simulink model "InvertedPendulumNoise"  (Simulink 7.5)
settings: Solver=ode45  SolverMode=SingleTasking  StartTime=0.0  StopTime=10  RelTol=1e-3  AbsTol=1e-6
values from neighbouring files (symbols this model uses):
  b = 0.1    [IP_BODE.m]    (also in IP_DIS.m; IP_FDT.m; IP_PID_1.m; IP_PID_2.m)
  g = 9.8    [IP_BODE.m]    (also in IP_DIS.m; IP_FDT.m; IP_PID_1.m; IP_PID_2.m)
  i = 0.006    [IP_BODE.m]    (also in IP_DIS.m; IP_FDT.m; IP_PID_1.m; IP_PID_2.m)
  l = 0.3    [IP_BODE.m]    (also in IP_DIS.m; IP_FDT.m; IP_PID_1.m; IP_PID_2.m)
  M = .5    (= 0.5)    [IP_BODE.m]    (also in IP_DIS.m; IP_FDT.m; IP_PID_1.m; IP_PID_2.m)
  m = 0.2    [IP_BODE.m]    (also in IP_DIS.m; IP_FDT.m; IP_PID_1.m; IP_PID_2.m)
libraries: simulink_need_slupdate x1
settings Model: Creator=neoben  LastModifiedBy=neoben
settings DataIOCC: LimitDataPoints=off
settings OptimizationCC: BlockReduction=off  BooleanDataType=off
settings DebuggingCC: SaveWithParameterizedLinksMsg=none  SignalResolutionControl=TryResolveAllWithWarning  SolverPrmCheckMsg=none  MultiTaskDSMMsg=warning  MultiTaskCondExecSysMsg=none  StrictBusMsg=None
settings HardwareCC: TargetUnknown=on
settings RTWCC: IncludeERTFirstTime=on

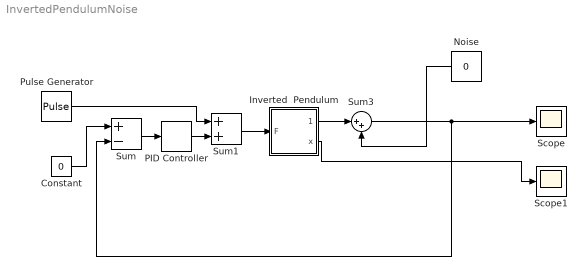
== system InvertedPendulumNoise ==
  Constant : Constant  Value=0
  Inverted  Pendulum : Subsystem
  Noise : Constant  Value=0  OutDataType=fixdt(1, 16)  OutScaling=2^0
  PID Controller : simulink_need_slupdate/PID Controller  SystemSampleTime=-1  P=100  I=1  D=20
  Pulse Generator : DiscretePulseGenerator  PulseType=Time based  Amplitude=1000  Period=10  PulseWidth=.01  PhaseDelay=0  SampleTime=1
  Scope : Scope
      settings: TickLabels=on  YMin=0  YMax=0.045  DataFormat=Array  MaxDataPoints=7000
  Scope1 : Scope
      settings: TickLabels=on  DataFormat=Array
  Sum : Sum  Inputs=+-  SaturateOnIntegerOverflow=on  InputSameDT=on  OutDataTypeStr=Inherit: Same as first input
  Sum1 : Sum  SaturateOnIntegerOverflow=on  InputSameDT=on  OutDataTypeStr=Inherit: Same as first input
  Sum3 : Sum  Inputs=|++  OutDataType=fixdt(1, 16)  OutScaling=2^0
  wires:
  Sum/1 -> PID Controller/1
  PID Controller/1 -> Sum1/2
  Inverted  Pendulum/1(Theta) -> Sum3/1
  Constant/1 -> Sum/1
  Pulse Generator/1 -> Sum1/1
  Sum1/1 -> Inverted  Pendulum/1(F)
  Inverted  Pendulum/2(x) -> Scope1/1
  Noise/1 -> Sum3/2
  Sum3/1 -> Sum/2, Scope/1

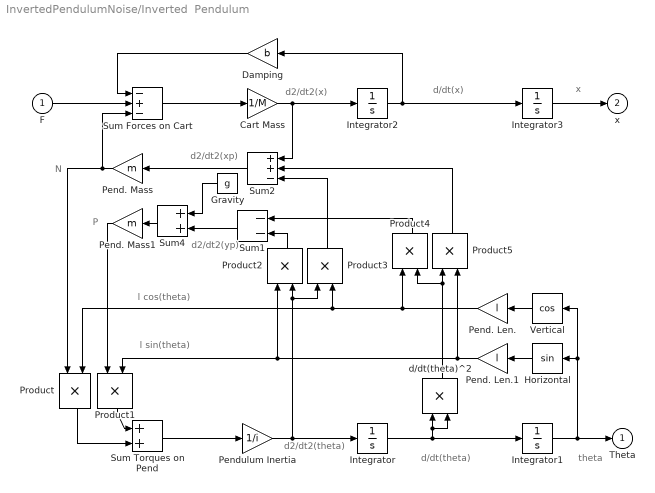
== system InvertedPendulumNoise/Inverted  Pendulum ==
  note: d2/dt2(xp)
  note: d2/dt2(yp)
  note: P
  note: N
  note: l sin(theta)
  note: l cos(theta)
  note: x
  note: d/dt(x)
  note: d2/dt2(x)
  note: d2/dt2(theta)
  note: d/dt(theta)
  note: theta
  F : Inport
  Cart Mass : Gain  Gain=1/M  SaturateOnIntegerOverflow=on  OutDataTypeStr=Inherit: Same as input  ParamDataTypeStr=Inherit: Same as input
  Damping : Gain  Gain=b  SaturateOnIntegerOverflow=on  OutDataTypeStr=Inherit: Same as input  ParamDataTypeStr=Inherit: Same as input
  Gravity : Constant  Value=g
  Horizontal : Trigonometry
  Integrator{,1..3} (4 alike) : Integrator
  Pend. Len. : Gain  Gain=l  SaturateOnIntegerOverflow=on  OutDataTypeStr=Inherit: Same as input  ParamDataTypeStr=Inherit: Same as input
  Pend. Len.1 : Gain  Gain=l  SaturateOnIntegerOverflow=on  OutDataTypeStr=Inherit: Same as input  ParamDataTypeStr=Inherit: Same as input
  Pend. Mass : Gain  Gain=m  SaturateOnIntegerOverflow=on  OutDataTypeStr=Inherit: Same as input  ParamDataTypeStr=Inherit: Same as input
  Pend. Mass1 : Gain  Gain=m  SaturateOnIntegerOverflow=on  OutDataTypeStr=Inherit: Same as input  ParamDataTypeStr=Inherit: Same as input
  Pendulum Inertia : Gain  Gain=1/i  SaturateOnIntegerOverflow=on  OutDataTypeStr=Inherit: Same as input  ParamDataTypeStr=Inherit: Same as input
  Product{,1..5} (6 alike) : Product  SaturateOnIntegerOverflow=on  RndMeth=Zero  InputSameDT=on  OutDataTypeStr=Inherit: Same as first input
  Sum Forces on Cart : Sum  Inputs=-+-  SaturateOnIntegerOverflow=on  InputSameDT=on  OutDataTypeStr=Inherit: Same as first input
  Sum Torques on Pend : Sum  SaturateOnIntegerOverflow=on  InputSameDT=on  OutDataTypeStr=Inherit: Same as first input
  Sum1 : Sum  Inputs=--  SaturateOnIntegerOverflow=on  InputSameDT=on  OutDataTypeStr=Inherit: Same as first input
  Sum2 : Sum  Inputs=++-  SaturateOnIntegerOverflow=on  InputSameDT=on  OutDataTypeStr=Inherit: Same as first input
  Sum4 : Sum  SaturateOnIntegerOverflow=on  InputSameDT=on  OutDataTypeStr=Inherit: Same as first input
  Vertical : Trigonometry  Operator=cos
  d/dt(theta)^2 : Product  SaturateOnIntegerOverflow=on  RndMeth=Zero  InputSameDT=on  OutDataTypeStr=Inherit: Same as first input
  Theta : Outport
  x : Outport  Port=2
  wires:
  Product2/1 -> Sum1/2
  Product3/1 -> Sum2/3
  Product4/1 -> Sum1/1
  Product5/1 -> Sum2/2
  Integrator/1 -> d/dt(theta)^2/2, d/dt(theta)^2/1, Integrator1/1
  Pend. Len.1/1 -> Product5/2, Product2/1, Product1/2
  Pend. Len./1 -> Product4/1, Product3/2, Product/2
  d/dt(theta)^2/1 -> Product4/2, Product5/1
  Pendulum Inertia/1 -> Product2/2, Product3/1, Integrator/1
  Cart Mass/1 -> Sum2/1, Integrator2/1
  Sum2/1 -> Pend. Mass/1
  Sum4/1 -> Pend. Mass1/1
  Sum1/1 -> Sum4/2
  Gravity/1 -> Sum4/1
  Pend. Mass/1 -> Sum Forces on Cart/3, Product/1
  Product1/1 -> Sum Torques on Pend/1
  Pend. Mass1/1 -> Product1/1
  Product/1 -> Sum Torques on Pend/2
  Integrator1/1 -> Vertical/1, Horizontal/1, Theta/1
  Vertical/1 -> Pend. Len./1
  Horizontal/1 -> Pend. Len.1/1
  F/1 -> Sum Forces on Cart/2
  Damping/1 -> Sum Forces on Cart/1
  Integrator2/1 -> Damping/1, Integrator3/1
  Sum Torques on Pend/1 -> Pendulum Inertia/1
  Sum Forces on Cart/1 -> Cart Mass/1
  Integrator3/1 -> x/1
